simulink model "main_RI_LIEKF"  (R2023a)
settings: Solver=FixedStepAuto  StartTime=0.0  StopTime=220  FixedStep=0.01  RelTol=1e-3
InitFcn:
  | initNavigation0612_AOA;
values from neighbouring files (symbols this model uses):
  CF_enable = 0    [initNavigation.m]
  dt = 0.01    [initNavigation.m]
  dtDelay = -0.03    [initNavigation.m]
  g0 = 9.795    [initNavigation.m]
  gam0_rad = 0/57.3    (= 0)    [initNavigation.m]
  H_sensor_type = 0    [initNavigation.m]
  KF_enable = 1    [initNavigation.m]
  P0 = diag([1*ones(3,1);0.01*ones(3,1);0.1*ones(3,1);0.001*ones(3,1);0.00001*ones(3,1)])    [initNavigation.m]
  P0_RIEKF = diag([1*ones(3,1);0.01*ones(3,1);0.1*ones(3,1);0.001*ones(3,1);0.00001*ones(3,1);      0.01*ones(3,1);[0;2;2]/57.3;[0.1;0.1;0.1]])^2    [initNavigation.m]
  pd0 = 0    [initNavigation.m]
  pe0 = 0    [initNavigation.m]
  phi0_rad = 0/57.3    (= 0)    [initNavigation.m]
  pn0 = 0    [initNavigation.m]
  psi = -178    [initNavigation.m]
  psi0_rad = 0/57.3    (= 0)    [initNavigation.m]
  state_dim = 24    [initNavigation.m]
  Time = 0:0.01:(size(traindata.AttackAngle,1) - 1)*0.01    [NNLiftCoefficientFit.m]
  vd0 = 0    [initNavigation.m]
  ve0 = 0    [initNavigation.m]
  vn0 = 0    [initNavigation.m]
undefined symbols (not defined in the file or in its folder): DiscIntNeverNeededParam, Discrete, INS_CONST, INS_EXPORT, INS_PARAM, magnitude, p, param, pInitialization, sys
libraries: simulink x69, simulink_extras x64, dspstat3 x56, sharedtransform x49, ctrlSharedLib x36, sharedTrackingLibrary x17, FMT_Model_Lib x13, matrix_library x12, deeplib x4, dspsolvers x4, vrlib x4, aerolibconvert2 x1
(part 6 of 22)

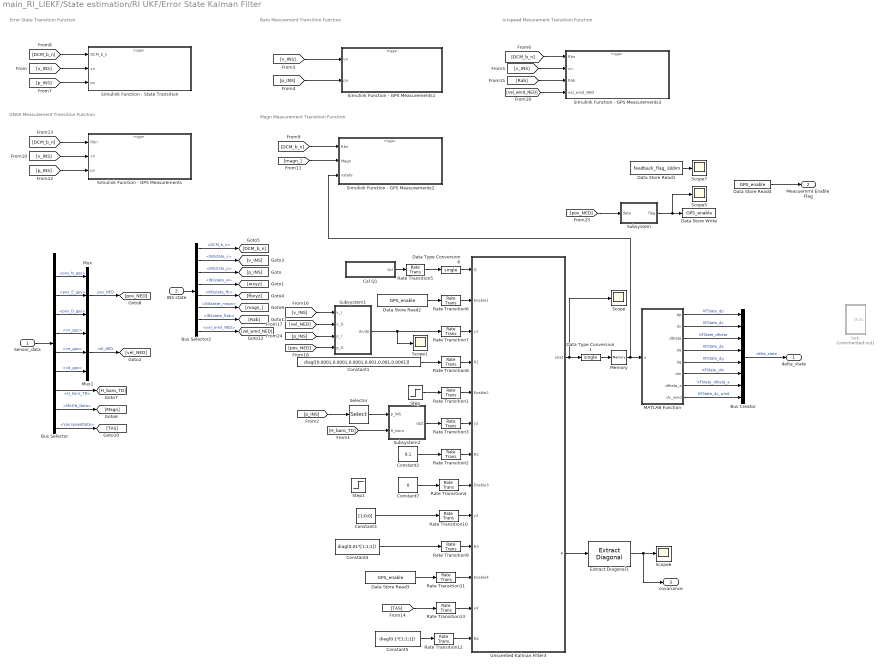
== system main_RI_LIEKF/State estimation/RI UKF/Error State Kalman Filter ==
  note: Error State Transition Function
  note: GNSS Measurement Transition Function
  note: Baro Mesurement Transition Function
  note: Magn Measurement Transition Function
  note: Airspeed Mesurement Transition Function
  Sensor_data : Inport
  INS state : Inport  Port=2
  Bus Creator : BusCreator  Inputs=8
  Bus Selector : BusSelector  OutputSignals=QGC_sensor_reinit,GPS_Data.pos_N_gps,GPS_Data.pos_E_gps,GPS_Data.pos_D_gps,GPS_Data.vn_gps,GPS_Data.ve_gps,GPS_Data.vd_gps,BARO_Data.H_baro_TD,MAGN_Data,VairspeedData
  Bus Selector2 : BusSelector  OutputSignals=RotationData.DCM_b_n,INSstate_v,INSstste_p,INSstate_w,INSstate_fb,INSstate_magn,INSstate_Rab,vel_wind_NED
  Cal Q1 : Subsystem
  Constant1 : Constant  Value=diag([0.0001,0.0001,0.0001,0.001,0.001,0.0001])  OutDataTypeStr=single
  Constant2 : Constant  Value=0.1  OutDataTypeStr=single
  Constant3 : Constant  Value=[1;0;0]  OutDataTypeStr=single
  Constant4 : Constant  Value=diag(0.01*[1;1;1])  OutDataTypeStr=single
  Constant5 : Constant  Value=diag(0.1*[1;1;1])  OutDataTypeStr=single
  Constant7 : Constant  Value=0  OutDataTypeStr=single
  Data Store Read1 : DataStoreRead  DataStoreName=feedback_flag_18dim  IndexOptions=Index vector (dialog)  Indices=1  OutputSizes=1
  Data Store Read2 : DataStoreRead  DataStoreName=GPS_enable  IndexOptions=Index vector (dialog)  Indices=1  OutputSizes=1
  Data Store Read3 : DataStoreRead  DataStoreName=GPS_enable  IndexOptions=Index vector (dialog)  Indices=1  OutputSizes=1
  Data Store Read4 : DataStoreRead  DataStoreName=GPS_enable  IndexOptions=Index vector (dialog)  Indices=1  OutputSizes=1
  Data Store Write : DataStoreWrite  DataStoreName=GPS_enable  IndexOptions=Index vector (dialog)  Indices=1  OutputSizes=1
  Data Type Conversion1 : DataTypeConversion  OutDataTypeStr=single  SaturateOnIntegerOverflow=off  RndMeth=Floor
  Data Type Conversion6 : DataTypeConversion  OutDataTypeStr=single  SaturateOnIntegerOverflow=off  RndMeth=Floor
  Extract Diagonal1 : matrix_library/Extract Diagonal
  MATLAB Function : MATLAB Function  TreatAsAtomicUnit=on
  Memory : Memory
  Mux : Mux  Inputs=3
  Mux1 : Mux  Inputs=3
  Rate Transition{1..13} (13 alike) : RateTransition  OutPortSampleTime=dt
  Scope{,1,5..7} (5 alike) : Scope
  Selector : Selector  InputPortWidth=3  IndexOptions=Index vector (dialog)  Indices=[3]  OutputSizes=1
  Simulink Function - GPS Measurements : Subsystem  TreatAsAtomicUnit=on
  Simulink Function - GPS Measurements1 : Subsystem  TreatAsAtomicUnit=on
  Simulink Function - GPS Measurements2 : Subsystem  TreatAsAtomicUnit=on
  Simulink Function - GPS Measurements3 : Subsystem  TreatAsAtomicUnit=on
  Simulink Function - State Transition : Subsystem  TreatAsAtomicUnit=on
  Step : Step  Time=5.01  OutDataTypeStr=single  SampleTime=0.01
  Step1 : Step  Time=5.01  OutDataTypeStr=single  SampleTime=0.01
  Subsystem : Subsystem
  Subsystem1 : Subsystem
  Subsystem2 : Subsystem
  Unscented Kalman Filter3 : Subsystem  mask(Unscented Kalman Filter){StateTransitionFcn=stateTransitionFcn_RIUKF, HasAdditiveProcessNoise=Nonadditive, ProcessNoise=1, HasTimeVaryingProcessNoise=on, HasStateTransitionFcnExtraArgument=0, InitialState=zeros(state_dim,1), InitialStateCovariance=P0_RIEKF, Alpha=1e-3, Beta=2, Kappa=0, MeasurementFcn1=GPSMeasurementFcn_RIUKF, HasMeasurementEnablePort1=on, HasAdditiveMeasurementNoise1=Nonadditive, MeasurementNoise1=1, HasTimeVaryingMeasurementNoise1=on, HasMeasurementFcnExtraArgument1=0, HasMeasurementWrapping1=off, MeasurementFcn2=BaroMeasurementFcn_RIUKF, HasMeasurementEnablePort2=on, HasAdditiveMeasurementNoise2=Nonadditive, MeasurementNoise2=1, HasTimeVaryingMeasurementNoise2=on, HasMeasurementFcnExtraArgument2=0, HasMeasurementWrapping2=off, MeasurementFcn3=MagnMeasurementFcn_RIUKF, HasMeasurementEnablePort3=on, HasAdditiveMeasurementNoise3=Nonadditive, MeasurementNoise3=1, HasTimeVaryingMeasurementNoise3=on, HasMeasurementFcnExtraArgument3=0, HasMeasurementWrapping3=off, MeasurementFcn4=AirspeedMeasurementFcn_RIUKF, HasMeasurementEnablePort4=on, HasAdditiveMeasurementNoise4=Nonadditive, MeasurementNoise4=1, HasTimeVaryingMeasurementNoise4=on, HasMeasurementFcnExtraArgument4=0, HasMeasurementWrapping4=off, MeasurementFcn5=myMeasurementFcn, HasMeasurementEnablePort5=off, HasAdditiveMeasurementNoise5=Additive, MeasurementNoise5=1, HasTimeVaryingMeasurementNoise5=off, HasMeasurementFcnExtraArgument5=0, HasMeasurementWrapping5=off, EnableMultirate=off, StateTransitionFcnSampleTime=1, MeasurementFcn1SampleTime=1, MeasurementFcn2SampleTime=1, MeasurementFcn3SampleTime=1, MeasurementFcn4SampleTime=1, MeasurementFcn5SampleTime=1, UseCurrentEstimator=on, OutputStateCovariance=on, DataType=single, SampleTime=0.01, NumberOfMeasurements=4}
      mask prompts: HasTimeVaryingProcessNoise "shared_tracking:blocks:maskPromptEKFUKFTimeVarying"; InitialState "shared_tracking:blocks:maskPromptEKFUKFInitialState"; InitialStateCovariance "shared_tracking:blocks:maskPromptEKFUKFInitialCovariance"; Alpha "shared_tracking:blocks:maskPromptUKFAlpha"; Beta "shared_tracking:blocks:maskPromptUKFBeta"; Kappa "shared_tracking:blocks:maskPromptUKFKappa"; HasMeasurementEnablePort1 "shared_tracking:blocks:maskPromptEnablePort"; HasTimeVaryingMeasurementNoise1 "shared_tracking:blocks:maskPromptEKFUKFTimeVarying"; HasMeasurementWrapping1 "shared_tracking:blocks:maskPromptEKFUKFMeasurementWrapping"; HasMeasurementEnablePort2 "shared_tracking:blocks:maskPromptEnablePort"; HasTimeVaryingMeasurementNoise2 "shared_tracking:blocks:maskPromptEKFUKFTimeVarying"; HasMeasurementWrapping2 "shared_tracking:blocks:maskPromptEKFUKFMeasurementWrapping"; HasMeasurementEnablePort3 "shared_tracking:blocks:maskPromptEnablePort"; HasTimeVaryingMeasurementNoise3 "shared_tracking:blocks:maskPromptEKFUKFTimeVarying"; HasMeasurementWrapping3 "shared_tracking:blocks:maskPromptEKFUKFMeasurementWrapping"; HasMeasurementEnablePort4 "shared_tracking:blocks:maskPromptEnablePort"; HasTimeVaryingMeasurementNoise4 "shared_tracking:blocks:maskPromptEKFUKFTimeVarying"; HasMeasurementWrapping4 "shared_tracking:blocks:maskPromptEKFUKFMeasurementWrapping"; HasMeasurementEnablePort5 "shared_tracking:blocks:maskPromptEnablePort"; HasTimeVaryingMeasurementNoise5 "shared_tracking:blocks:maskPromptEKFUKFTimeVarying"; HasMeasurementWrapping5 "shared_tracking:blocks:maskPromptEKFUKFMeasurementWrapping"; EnableMultirate "shared_tracking:blocks:maskPromptEnableMultirate"; StateTransitionFcnSampleTime "shared_tracking:blocks:maskPromptStateTransition"; MeasurementFcn1SampleTime "shared_tracking:blocks:maskPromptMeasurement1"; MeasurementFcn2SampleTime "shared_tracking:blocks:maskPromptMeasurement2"; MeasurementFcn3SampleTime "shared_tracking:blocks:maskPromptMeasurement3"; MeasurementFcn4SampleTime "shared_tracking:blocks:maskPromptMeasurement4"; MeasurementFcn5SampleTime "shared_tracking:blocks:maskPromptMeasurement5"; UseCurrentEstimator "shared_tracking:blocks:maskPromptUseCurrentEstimator"; OutputStateCovariance "shared_tracking:blocks:maskPromptOutputStateCovariance"; DataType "shared_tracking:blocks:maskPromptDataType"; SampleTime "shared_tracking:blocks:maskPromptSampleTime"
      mask help: shared_tracking:blocks:maskPromptUKFDescription
      mask init:
      | matlabshared.tracking.internal.blocks.maskInitializationScriptUKF
      mask Help: eval('matlabshared.tracking.internal.blocks.controlIdentLaunchDocPage(''UKF'')')
      mask TypeOptions HasAdditiveProcessNoise: shared_tracking:blocks:maskPromptEKFUKFAdditiveNoise | shared_tracking:blocks:maskPromptEKFUKFNonAdditiveNoise
      mask Callback HasTimeVaryingProcessNoise: matlabshared.tracking.internal.blocks.dialogCallbacksEKFUKFPF(gcbh,'checkboxIsCovarianceTimeVarying','HasTimeVaryingProcessNoise','ProcessNoise')
      mask TypeOptions HasAdditiveMeasurementNoise1: shared_tracking:blocks:maskPromptEKFUKFAdditiveNoise | shared_tracking:blocks:maskPromptEKFUKFNonAdditiveNoise
      mask Callback HasTimeVaryingMeasurementNoise1: matlabshared.tracking.internal.blocks.dialogCallbacksEKFUKFPF(gcbh,'checkboxIsCovarianceTimeVarying','HasTimeVaryingMeasurementNoise1','MeasurementNoise1')
      mask TypeOptions HasAdditiveMeasurementNoise2: shared_tracking:blocks:maskPromptEKFUKFAdditiveNoise | shared_tracking:blocks:maskPromptEKFUKFNonAdditiveNoise
      mask Callback HasTimeVaryingMeasurementNoise2: matlabshared.tracking.internal.blocks.dialogCallbacksEKFUKFPF(gcbh,'checkboxIsCovarianceTimeVarying','HasTimeVaryingMeasurementNoise2','MeasurementNoise2')
      mask TypeOptions HasAdditiveMeasurementNoise3: shared_tracking:blocks:maskPromptEKFUKFAdditiveNoise | shared_tracking:blocks:maskPromptEKFUKFNonAdditiveNoise
      mask Callback HasTimeVaryingMeasurementNoise3: matlabshared.tracking.internal.blocks.dialogCallbacksEKFUKFPF(gcbh,'checkboxIsCovarianceTimeVarying','HasTimeVaryingMeasurementNoise3','MeasurementNoise3')
      mask TypeOptions HasAdditiveMeasurementNoise4: shared_tracking:blocks:maskPromptEKFUKFAdditiveNoise | shared_tracking:blocks:maskPromptEKFUKFNonAdditiveNoise
      mask Callback HasTimeVaryingMeasurementNoise4: matlabshared.tracking.internal.blocks.dialogCallbacksEKFUKFPF(gcbh,'checkboxIsCovarianceTimeVarying','HasTimeVaryingMeasurementNoise4','MeasurementNoise4')
      mask TypeOptions HasAdditiveMeasurementNoise5: shared_tracking:blocks:maskPromptEKFUKFAdditiveNoise | shared_tracking:blocks:maskPromptEKFUKFNonAdditiveNoise
      mask Callback HasTimeVaryingMeasurementNoise5: matlabshared.tracking.internal.blocks.dialogCallbacksEKFUKFPF(gcbh,'checkboxIsCovarianceTimeVarying','HasTimeVaryingMeasurementNoise5','MeasurementNoise5')
      mask Callback EnableMultirate: matlabshared.tracking.internal.blocks.dialogCallbacksEKFUKFPF(gcbh,'checkBoxHasMultirate')
      mask TypeOptions DataType: shared_tracking:blocks:maskPromptDouble | shared_tracking:blocks:maskPromptSingle
      mask Callback NumberOfMeasurements: matlabshared.tracking.internal.blocks.dialogCallbacksEKFUKFPF(gcbh,'editboxNumberOfMeasurements','MeasurementFcn');
      mask DialogControl DescGroupVar Prompt: shared_tracking:blocks:maskPromptUKFTitle
      mask DialogControl TabSystemModel Prompt: shared_tracking:blocks:maskPromptSystemModel
      mask DialogControl GroupStateTransition Prompt: shared_tracking:blocks:maskPromptStateTransition
      mask DialogControl StateTransitionFunctionText Prompt: shared_tracking:blocks:maskPromptFunction
      mask DialogControl ProcessNoiseText Prompt: shared_tracking:blocks:maskPromptEKFUKFProcessNoise
      mask DialogControl ProcessNoiseCovarianceText Prompt: shared_tracking:blocks:maskPromptCovariance
      mask DialogControl HasTimeVaryingProcessNoise Prompt: Time-varying
      mask DialogControl InitializationContainer Prompt: shared_tracking:blocks:maskPromptInitialization
      mask DialogControl InitialState Prompt: Initial state:
      mask DialogControl InitialStateCovariance Prompt: Initial covariance:
      mask DialogControl ContainerUTParameters Prompt: shared_tracking:blocks:maskPromptUKFUTParameters
      mask DialogControl Alpha Prompt: Alpha:
      mask DialogControl Beta Prompt: Beta:
      mask DialogControl Kappa Prompt: Kappa:
      mask DialogControl GroupMeasurement1 Prompt: shared_tracking:blocks:maskPromptMeasurement1
      mask DialogControl MeasurementFunction1Text Prompt: shared_tracking:blocks:maskPromptFunction
      mask DialogControl HasMeasurementEnablePort1 Prompt: Add Enable port
      mask DialogControl MeasurementNoiseText1 Prompt: shared_tracking:blocks:maskPromptEKFUKFMeasurementNoise
      mask DialogControl MeasurementNoiseCovarianceText1 Prompt: shared_tracking:blocks:maskPromptCovariance
      mask DialogControl HasTimeVaryingMeasurementNoise1 Prompt: Time-varying
      mask DialogControl HasMeasurementWrapping1 Prompt: Has measurement wrapping
      mask DialogControl GroupMeasurement2 Prompt: shared_tracking:blocks:maskPromptMeasurement2
      mask DialogControl MeasurementFunction2Text Prompt: shared_tracking:blocks:maskPromptFunction
      mask DialogControl HasMeasurementEnablePort2 Prompt: Add Enable port
      mask DialogControl MeasurementNoiseText2 Prompt: shared_tracking:blocks:maskPromptEKFUKFMeasurementNoise
      mask DialogControl MeasurementNoiseCovarianceText2 Prompt: shared_tracking:blocks:maskPromptCovariance
      mask DialogControl HasTimeVaryingMeasurementNoise2 Prompt: Time-varying
      mask DialogControl HasMeasurementWrapping2 Prompt: Has measurement wrapping
      mask DialogControl GroupMeasurement3 Prompt: shared_tracking:blocks:maskPromptMeasurement3
      mask DialogControl MeasurementFunction3Text Prompt: shared_tracking:blocks:maskPromptFunction
      mask DialogControl HasMeasurementEnablePort3 Prompt: Add Enable port
      mask DialogControl MeasurementNoiseText3 Prompt: shared_tracking:blocks:maskPromptEKFUKFMeasurementNoise
      mask DialogControl MeasurementNoiseCovarianceText3 Prompt: shared_tracking:blocks:maskPromptCovariance
      mask DialogControl HasTimeVaryingMeasurementNoise3 Prompt: Time-varying
      mask DialogControl HasMeasurementWrapping3 Prompt: Has measurement wrapping
      mask DialogControl GroupMeasurement4 Prompt: shared_tracking:blocks:maskPromptMeasurement4
      mask DialogControl MeasurementFunction4Text Prompt: shared_tracking:blocks:maskPromptFunction
      mask DialogControl HasMeasurementEnablePort4 Prompt: Add Enable port
      mask DialogControl MeasurementNoiseText4 Prompt: shared_tracking:blocks:maskPromptEKFUKFMeasurementNoise
      mask DialogControl MeasurementNoiseCovarianceText4 Prompt: shared_tracking:blocks:maskPromptCovariance
      mask DialogControl HasTimeVaryingMeasurementNoise4 Prompt: Time-varying
      mask DialogControl HasMeasurementWrapping4 Prompt: Has measurement wrapping
      mask DialogControl GroupMeasurement5 Prompt: shared_tracking:blocks:maskPromptMeasurement5
      mask DialogControl MeasurementFunction5Text Prompt: shared_tracking:blocks:maskPromptFunction
      mask DialogControl HasMeasurementEnablePort5 Prompt: Add Enable port
      mask DialogControl MeasurementNoiseText5 Prompt: shared_tracking:blocks:maskPromptEKFUKFMeasurementNoise
      mask DialogControl MeasurementNoiseCovarianceText5 Prompt: shared_tracking:blocks:maskPromptCovariance
      mask DialogControl HasTimeVaryingMeasurementNoise5 Prompt: Time-varying
      mask DialogControl HasMeasurementWrapping5 Prompt: Has measurement wrapping
      mask DialogControl AddMeasurement Prompt: shared_tracking:blocks:maskPromptAddMeasurement
      mask DialogControl AddMeasurement Callback: matlabshared.tracking.internal.blocks.dialogCallbacksEKFUKFPF(gcbh,'buttonAddMeasurement','MeasurementFcn');
      mask DialogControl RemoveMeasurement Prompt: shared_tracking:blocks:maskPromptRemoveMeasurement
      mask DialogControl RemoveMeasurement Callback: matlabshared.tracking.internal.blocks.dialogCallbacksEKFUKFPF(gcbh,'buttonRemoveMeasurement','MeasurementFcn');
      mask DialogControl TabMultirate Prompt: shared_tracking:blocks:maskPromptEKFUKFMultirate
      mask DialogControl GroupMultirate Prompt: shared_tracking:blocks:maskPromptEKFUKFMultirate
      mask DialogControl EnableMultirate Prompt: Enable multirate operation
      mask DialogControl GroupMultirateSampleTimes Prompt: shared_tracking:blocks:maskPromptSampleTimeNoInheritance
      mask DialogControl StateTransitionFcnSampleTime Prompt: State Transition
      mask DialogControl MeasurementFcn1SampleTime Prompt: Measurement 1
      mask DialogControl MeasurementFcn2SampleTime Prompt: Measurement 2
      mask DialogControl MeasurementFcn3SampleTime Prompt: Measurement 3
      mask DialogControl MeasurementFcn4SampleTime Prompt: Measurement 4
      mask DialogControl MeasurementFcn5SampleTime Prompt: Measurement 5
      mask DialogControl ContainerSettings Prompt: shared_tracking:blocks:maskPromptEKFUKFSettings
      mask DialogControl UseCurrentEstimator Prompt: Use the current measurements to improve state estimates
      mask DialogControl OutputStateCovariance Prompt: Output state estimation error covariance
      mask DialogControl DataType Prompt: Data type:
      mask DialogControl SampleTime Prompt: Sample time:
  bak : Subsystem  Commented=on
  delta_state : Outport
  Measuemrnt Enable Flag : Outport  Port=2
  covariance : Outport  Port=3
  wires:
  Bus Creator/1 -> delta_state/1  "delta_state"
  Data Type Conversion1/1 -> Memory/1
  MATLAB Function/5(dg) -> Bus Creator/5  "KFState_dg"
  MATLAB Function/2(dv) -> Bus Creator/2  "KFState_dv"
  MATLAB Function/4(da) -> Bus Creator/4  "KFState_da"
  Bus Selector2/3 -> [p_INS]  "<INSstste_p>"
  Bus Selector2/1 -> [DCM_b_n]  "<DCM_b_n>"
  Bus Selector2/5 -> [fbxyz]  "<INSstate_fb>"
  Bus Selector2/4 -> [wxyz]  "<INSstate_w>"
  INS state/1 -> Bus Selector2/1
  Bus Selector/4 -> Mux/3  "<pos_D_gps>"
  Bus Selector/2 -> Mux/1  "<pos_N_gps>"
  Bus Selector/3 -> Mux/2  "<pos_E_gps>"
  Bus Selector/7 -> Mux1/3  "<vd_gps>"
  Bus Selector/5 -> Mux1/1  "<vn_gps>"
  Mux1/1 -> [vel_NED]  "vel_NED"
  Sensor_data/1 -> Bus Selector/1
  Bus Selector/6 -> Mux1/2  "<ve_gps>"
  Data Store Read1/1 -> Scope7/1
  [pos_NED] -> Subsystem/1(data)
  Subsystem/1(flag) -> Data Store Write/1, Scope5/1
  Unscented Kalman Filter3/1(xhat) -> Scope/1, Data Type Conversion1/1
  MATLAB Function/1(dp) -> Bus Creator/1  "KFState_dp"
  MATLAB Function/3(dtheta) -> Bus Creator/3  "KFState_dtheta"
  [DCM_b_n] -> Simulink Function - State Transition/1(DCM_b_n)
  Constant1/1 -> Rate Transition8/1
  Unscented Kalman Filter3/2(P) -> Extract Diagonal1/1
  Extract Diagonal1/1 -> covariance/1, Scope6/1
  Rate Transition6/1 -> Unscented Kalman Filter3/2(Enable1)
  Rate Transition7/1 -> Unscented Kalman Filter3/3(y1)
  Rate Transition8/1 -> Unscented Kalman Filter3/4(R1)
  Cal Q1/1(Qd) -> Rate Transition5/1
  Rate Transition5/1 -> Data Type Conversion6/1
  Data Type Conversion6/1 -> Unscented Kalman Filter3/1(Q)
  Bus Selector2/2 -> [v_INS]  "<INSstate_v>"
  Mux/1 -> [pos_NED]  "pos_NED"
  Data Store Read4/1 -> Measuemrnt Enable Flag/1
  [v_INS] -> Simulink Function - State Transition/2(vn)
  [p_INS] -> Simulink Function - State Transition/3(pn)
  Subsystem1/1(dv/dp) -> Scope1/1, Rate Transition7/1
  [v_INS] -> Subsystem1/1(v_I)
  [vel_NED] -> Subsystem1/2(v_G)
  [p_INS] -> Subsystem1/3(p_I)
  [pos_NED] -> Subsystem1/4(p_G)
  [DCM_b_n] -> Simulink Function - GPS Measurements/1(Rbn)
  [v_INS] -> Simulink Function - GPS Measurements/2(vn)
  [p_INS] -> Simulink Function - GPS Measurements/3(pn)
  Bus Selector/8 -> [H_baro_TD]  "<H_baro_TD>"
  Rate Transition1/1 -> Unscented Kalman Filter3/5(Enable2)
  Step/1 -> Rate Transition1/1
  Rate Transition2/1 -> Unscented Kalman Filter3/7(R2)
  Constant2/1 -> Rate Transition2/1
  [p_INS] -> Simulink Function - GPS Measurements1/2(pn)
  [v_INS] -> Simulink Function - GPS Measurements1/1(vn)
  Rate Transition3/1 -> Unscented Kalman Filter3/6(y2)
  [p_INS] -> Selector/1
  Subsystem2/1(dpZ) -> Rate Transition3/1
  Selector/1 -> Subsystem2/1(p_INS)
  [H_baro_TD] -> Subsystem2/2(H_baro)
  Bus Selector/9 -> [Magn]  "<MAGN_Data>"
  Rate Transition4/1 -> Unscented Kalman Filter3/8(Enable3)
  Constant3/1 -> Rate Transition10/1
  Constant4/1 -> Rate Transition9/1
  Rate Transition9/1 -> Unscented Kalman Filter3/10(R3)
  Rate Transition10/1 -> Unscented Kalman Filter3/9(y3)
  [magn_] -> Simulink Function - GPS Measurements2/2(Magn)
  Data Store Read2/1 -> Rate Transition6/1
  [DCM_b_n] -> Simulink Function - GPS Measurements2/1(Rbn)
  MATLAB Function/6(dm) -> Bus Creator/6  "KFState_dm"
  Bus Selector2/6 -> [magn_]  "<INSstate_magn>"
  [DCM_b_n] -> Simulink Function - GPS Measurements3/1(Rbn)
  [v_INS] -> Simulink Function - GPS Measurements3/2(vn)
  Memory/1 -> Simulink Function - GPS Measurements2/3(xstate), MATLAB Function/1(u)
  Rate Transition11/1 -> Unscented Kalman Filter3/11(Enable4)
  Bus Selector/10 -> [TAS]  "<VairspeedData>"
  [TAS] -> Rate Transition13/1
  MATLAB Function/7(dtheta_a) -> Bus Creator/7  "KFState_dtheta_a"
  MATLAB Function/8(dv_wind) -> Bus Creator/8  "KFState_dv_wind"
  Constant5/1 -> Rate Transition12/1
  Rate Transition12/1 -> Unscented Kalman Filter3/13(R4)
  Bus Selector2/7 -> [Rab]  "<INSstate_Rab>"
  [Rab] -> Simulink Function - GPS Measurements3/3(Rab)
  Bus Selector2/8 -> [vel_wind_NED]  "<vel_wind_NED>"
  [vel_wind_NED] -> Simulink Function - GPS Measurements3/4(vel_wind_NED)
  Rate Transition13/1 -> Unscented Kalman Filter3/12(y4)
  Data Store Read3/1 -> Rate Transition11/1
  Constant7/1 -> Rate Transition4/1

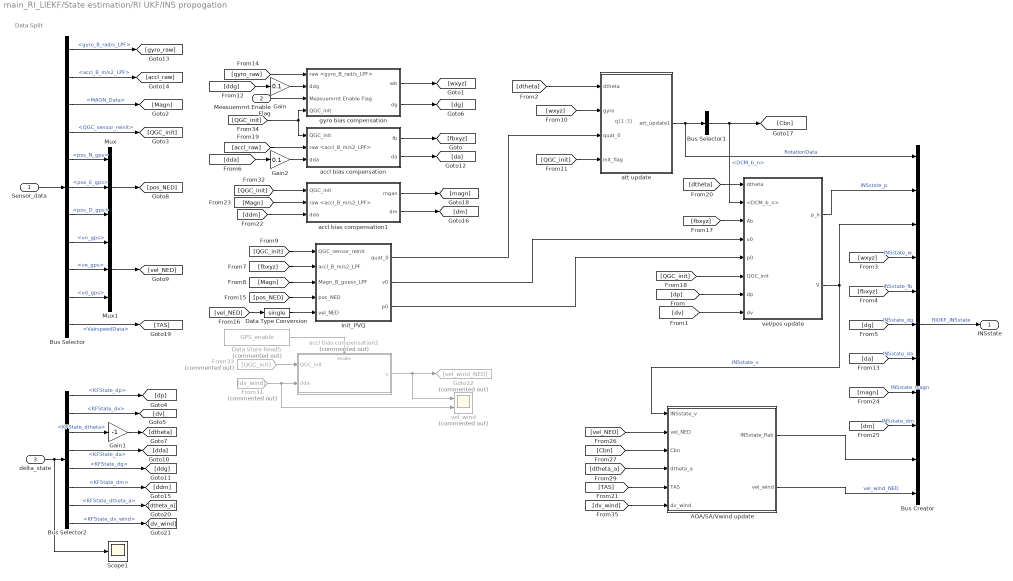
== system main_RI_LIEKF/State estimation/RI UKF/INS propogation ==
  note: Data Split
  note: q(1:3)
  Sensor_data : Inport
  Measuemrnt Enable Flag : Inport  Port=2
  delta_state : Inport  Port=3
  AOA/SA/Vwind update : Subsystem
  Bus Creator : BusCreator  Inputs=11
  Bus Selector : BusSelector  OutputSignals=IMU_Data.gyro_B_rad/s_LPF,IMU_Data.accl_B_m/s2_LPF,MAGN_Data,QGC_sensor_reinit,GPS_Data.pos_N_gps,GPS_Data.pos_E_gps,GPS_Data.pos_D_gps,GPS_Data.vn_gps,GPS_Data.ve_gps,GPS_Data.vd_gps,VairspeedData
  Bus Selector1 : BusSelector  OutputSignals=DCM_b_n
  Bus Selector2 : BusSelector  OutputSignals=KFState_dp,KFState_dv,KFState_dtheta,KFState_da,KFState_dg,KFState_dm,KFState_dtheta_a,KFState_dv_wind
  Data Store Read5 : DataStoreRead  Commented=on  DataStoreName=GPS_enable  IndexOptions=Index vector (dialog)  Indices=1  OutputSizes=1
  Data Type Conversion : DataTypeConversion  OutDataTypeStr=single  SaturateOnIntegerOverflow=off  RndMeth=Floor
  From31 : From  Commented=on  GotoTag=dv_wind
  From33 : From  Commented=on  GotoTag=QGC_init
  Gain : Gain  Gain=0.1
  Gain1 : Gain  Gain=-1
  Gain2 : Gain  Gain=0.1
  Goto22 : Goto  Commented=on  GotoTag=vel_wind_NED
  Init_PVQ : Subsystem
  Mux : Mux  Inputs=3
  Mux1 : Mux  Inputs=3
  Scope1 : Scope
  accl bias compensation : Subsystem
  accl bias compensation1 : Subsystem
  accl bias compensation2 : Subsystem  Commented=on
  att update : Subsystem
  gyro bias compensation : Subsystem
  vel/pos update : Subsystem
  vel_wind : Scope  Commented=on  NumInputPorts=2
  INSstate : Outport
  wires:
  Bus Selector/2 -> [accl_raw]  "<accl_B_m/s2_LPF>"
  [accl_raw] -> accl bias compensation/2(raw <accl_B_m/s2_LPF>)
  [gyro_raw] -> gyro bias compensation/1(raw <gyro_B_rad/s_LPF>)
  Bus Selector2/5 -> [ddg]  "<KFState_dg>"
  Bus Selector2/4 -> [dda]  "<KFState_da>"
  Bus Selector2/3 -> Gain1/1  "<KFState_dtheta>"
  Bus Selector2/2 -> [dv]  "<KFState_dv>"
  Bus Selector2/1 -> [dp]  "<KFState_dp>"
  delta_state/1 -> Scope1/1, Bus Selector2/1
  [da] -> Bus Creator/7  "INSstate_da"
  [dg] -> Bus Creator/6  "INSstate_dg"
  gyro bias compensation/2(dg) -> [dg]
  gyro bias compensation/1(wb) -> [wxyz]
  Measuemrnt Enable Flag/1 -> gyro bias compensation/3(Measuemrnt Enable Flag)
  accl bias compensation/2(da) -> [da]
  accl bias compensation/1(fb) -> [fbxyz]
  Bus Creator/1 -> INSstate/1  "RIUKF_INSstate"
  att update/1(att_update1) -> Bus Creator/1, Bus Selector1/1  "RotationData"
  [fbxyz] -> Bus Creator/5  "INSstate_fb"
  [wxyz] -> Bus Creator/4  "INSstate_w"
  vel/pos update/1(p_k) -> Bus Creator/2  "INSstste_p"
  [QGC_init] -> Init_PVQ/1(QGC_sensor_reinit)
  [dv] -> vel/pos update/8(dv)
  vel/pos update/2(V) -> AOA/SA/Vwind update/1(INSstate_v), Bus Creator/3  "INSstate_v"
  Bus Selector1/1 -> vel/pos update/2(<DCM_b_n>), [Cbn]  "<DCM_b_n>"
  Bus Selector/1 -> [gyro_raw]  "<gyro_B_rad/s_LPF>"
  Bus Selector/4 -> [QGC_init]  "<QGC_sensor_reinit>"
  [Magn] -> Init_PVQ/3(Magn_B_guess_LPF)
  [dp] -> vel/pos update/7(dp)
  Data Type Conversion/1 -> Init_PVQ/5(vel_NED)
  [pos_NED] -> Init_PVQ/4(pos_NED)
  [QGC_init] -> vel/pos update/6(QGC_init)
  Bus Selector/9 -> Mux1/2  "<ve_gps>"
  Init_PVQ/3(p0) -> vel/pos update/5(p0)
  Init_PVQ/2(v0) -> vel/pos update/4(v0)
  [fbxyz] -> Init_PVQ/2(accl_B_m/s2_LPF)
  Sensor_data/1 -> Bus Selector/1
  Mux1/1 -> [vel_NED]
  Bus Selector/3 -> [Magn]  "<MAGN_Data>"
  Bus Selector/6 -> Mux/2  "<pos_E_gps>"
  [wxyz] -> att update/2(gyro)
  Bus Selector/5 -> Mux/1  "<pos_N_gps>"
  Bus Selector/8 -> Mux1/1  "<vn_gps>"
  Bus Selector/7 -> Mux/3  "<pos_D_gps>"
  [vel_NED] -> Data Type Conversion/1
  Bus Selector/10 -> Mux1/3  "<vd_gps>"
  [QGC_init] -> att update/4(init_flag)
  [fbxyz] -> vel/pos update/3(Ab)
  Init_PVQ/1(quat_0) -> att update/3(quat_0)
  Mux/1 -> [pos_NED]
  [dtheta] -> vel/pos update/1(dtheta)
  [QGC_init] -> gyro bias compensation/4(QGC_init), accl bias compensation/1(QGC_init)
  Gain1/1 -> [dtheta]
  [ddg] -> Gain/1
  [dda] -> Gain2/1
  [dtheta] -> att update/1(dtheta)
  Bus Selector2/6 -> [ddm]  "<KFState_dm>"
  [Magn] -> accl bias compensation1/2(raw <accl_B_m/s2_LPF>)
  [ddm] -> accl bias compensation1/3(dda)
  accl bias compensation1/2(dm) -> [dm]
  accl bias compensation1/1(mgan) -> [magn]
  [magn] -> Bus Creator/8  "INSstate_magn"
  [dm] -> Bus Creator/9  "INSstate_dm"
  Bus Selector/11 -> [TAS]  "<VairspeedData>"
  Bus Selector2/7 -> [dtheta_a]  "<KFState_dtheta_a>"
  Bus Selector2/8 -> [dv_wind]  "<KFState_dv_wind>"
  From31/1 -> vel_wind/2, accl bias compensation2/2(dda)
  [QGC_init] -> accl bias compensation1/1(QGC_init)
  From33/1 -> accl bias compensation2/1(QGC_init)
  accl bias compensation2/1(v) -> vel_wind/1, Goto22/1
  AOA/SA/Vwind update/2(vel_wind) -> Bus Creator/11  "vel_wind_NED"
  [vel_NED] -> AOA/SA/Vwind update/2(vel_NED)
  [Cbn] -> AOA/SA/Vwind update/3(Cbn)
  [dtheta_a] -> AOA/SA/Vwind update/4(dtheta_a)
  AOA/SA/Vwind update/1(INSstate_Rab) -> Bus Creator/10
  Data Store Read5/1 -> accl bias compensation2/Enable
  [TAS] -> AOA/SA/Vwind update/5(TAS)
  [dv_wind] -> AOA/SA/Vwind update/6(dv_wind)
  Gain/1 -> gyro bias compensation/2(ddg)
  Gain2/1 -> accl bias compensation/3(dda)

== system main_RI_LIEKF/State estimation/bak1/Bus_Constructor ==
  INSstate : Inport
  Bus Creator : BusCreator  Inputs=1
  Bus Creator2 : BusCreator  Inputs=6
  Bus Selector : BusSelector  OutputSignals=RotationData.DCM_b_n,INSstate_v,INSstste_p,INSstate_dg,INSstate_da
  Demux : Demux  Outputs=3
  Demux1 : Demux  Outputs=3
  Scope : Scope  NumInputPorts=2
  TranslationData : Outport
  RotationData : Outport  Port=2
  wires:
  Demux/1 -> Bus Creator2/1  "vn_m/s"
  Bus Selector/2 -> Demux/1  "<INSstate_v>"
  Demux1/3 -> Bus Creator2/6  "H_m"
  Demux1/1 -> Bus Creator2/4  "pn_m"
  Demux1/2 -> Bus Creator2/5  "pe_m"
  Demux/3 -> Bus Creator2/3  "vd_m/s"
  Bus Creator2/1 -> TranslationData/1
  Demux/2 -> Bus Creator2/2  "ve_m/s"
  INSstate/1 -> Bus Selector/1
  Bus Selector/1 -> Bus Creator/1  "<DCM_b_n>"
  Bus Creator/1 -> RotationData/1
  Bus Selector/3 -> Demux1/1  "<INSstste_p>"
  Bus Selector/4 -> Scope/1  "<INSstate_dg>"
  Bus Selector/5 -> Scope/2  "<INSstate_da>"
